simulink model "gazebo_cosimulation_waypoint_follower"  (R2023b)
settings: Solver=VariableStepAuto  StartTime=0.0  StopTime=10.0  RelTol=1e-3
undefined symbols (not defined in the file): center_cylinder, quadcopter, rotor_1, rotor_2, rotor_3, rotor_4
libraries: robotgazebolib x11, simulink x1
settings Model: Creator=rakshan  LastModifiedBy=rakshan

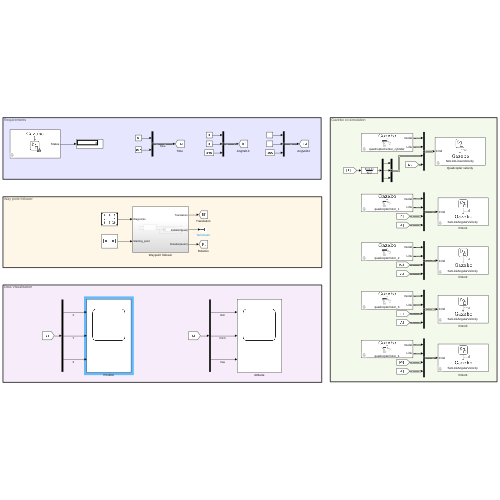
[thumbnail: Simulink's stored preview of the top-level diagram]
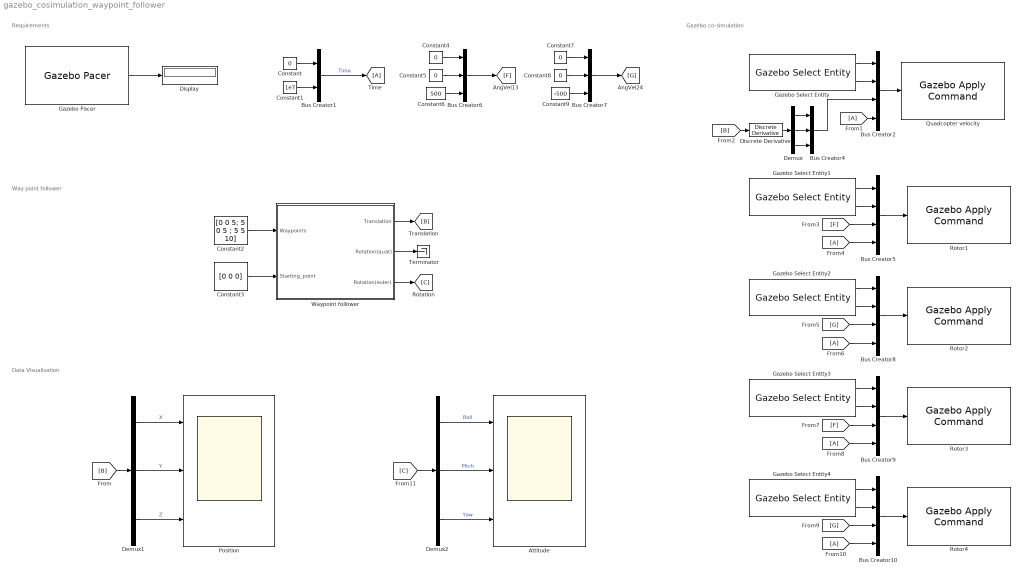
== system gazebo_cosimulation_waypoint_follower ==
  note: Data Visualisation
  note: Way point follower
  note: Requirements
  note: Gazebo co-simulation
  Attitude : Scope  NumInputPorts=3
  Bus Creator1 : BusCreator  Inputs=2  OutDataTypeStr=Bus: Gazebo_SL_Bus_gazebo_msgs_Time  NonVirtualBus=on
      settings: InheritFromInputs=off
  Bus Creator{5,8..10} (4 alike) : BusCreator  Inputs=4  OutDataTypeStr=Bus: Gazebo_SL_Bus_gazebo_msgs_SetLinkAngularVelocity  NonVirtualBus=on
      settings: InheritFromInputs=off
  Bus Creator2 : BusCreator  Inputs=4  OutDataTypeStr=Bus: Gazebo_SL_Bus_gazebo_msgs_SetLinkLinearVelocity  NonVirtualBus=on
      settings: InheritFromInputs=off
  Bus Creator4 : BusCreator  Inputs=3  OutDataTypeStr=Bus: Gazebo_SL_Bus_gazebo_msgs_Point  NonVirtualBus=on
      settings: InheritFromInputs=off
  Bus Creator6 : BusCreator  Inputs=3  OutDataTypeStr=Bus: Gazebo_SL_Bus_gazebo_msgs_Point  NonVirtualBus=on
      settings: InheritFromInputs=off
  Bus Creator7 : BusCreator  Inputs=3  OutDataTypeStr=Bus: Gazebo_SL_Bus_gazebo_msgs_Point  NonVirtualBus=on
      settings: InheritFromInputs=off
  Constant{,4..5,7..8} (5 alike) : Constant  Value=0
  Constant1 : Constant  Value=1e7
  Constant2 : Constant  Value=[0 0 5; 5 0 5 ; 5 5 10]
  Constant3 : Constant  Value=[0 0 0]  VectorParams1D=off
  Constant6 : Constant  Value=500
  Constant9 : Constant  Value=-500
  Demux : Demux  Outputs=3
  Demux1 : Demux  Outputs=3
  Demux2 : Demux  Outputs=3
  Discrete Derivative : simulink/Discrete/Discrete Derivative  gainval=1.0  ICPrevScaledInput=0.0  OutMin=[]  OutMax=[]  OutDataType=fixdt(1, 16)  OutScaling=2^-10  DoSatur=off
  Display : Display
  From{1,4,6,8,10} (5 alike) : From
  Gazebo Pacer : robotgazebolib/Gazebo Pacer  ResetBehavior=Reset Gazebo simulation time  SampleTime=0.001
  Gazebo Select Entity : robotgazebolib/Gazebo Select Entity  modelElemName=quadcopter/center_cylinder  outputArraySize=128  OutputLabel=Link  SelectType=Link
  Gazebo Select Entity1 : robotgazebolib/Gazebo Select Entity  modelElemName=quadcopter/rotor_1  outputArraySize=128  OutputLabel=Link  SelectType=Link
  Gazebo Select Entity2 : robotgazebolib/Gazebo Select Entity  modelElemName=quadcopter/rotor_2  outputArraySize=128  OutputLabel=Link  SelectType=Link
  Gazebo Select Entity3 : robotgazebolib/Gazebo Select Entity  modelElemName=quadcopter/rotor_3  outputArraySize=128  OutputLabel=Link  SelectType=Link
  Gazebo Select Entity4 : robotgazebolib/Gazebo Select Entity  modelElemName=quadcopter/rotor_4  outputArraySize=128  OutputLabel=Link  SelectType=Link
  Position : Scope  NumInputPorts=3
  Quadcopter velocity : robotgazebolib/Gazebo Apply Command  cmdType=SetLinkLinearVelocity  sampleTime=0.001
  Rotor{1..4} (4 alike) : robotgazebolib/Gazebo Apply Command  cmdType=SetLinkAngularVelocity  sampleTime=0.001
  Terminator : Terminator
  Time : Goto
  Waypoint follower : Subsystem
  wires:
  Constant3/1 -> Waypoint follower/2(Starting_point)
  Constant2/1 -> Waypoint follower/1(Waypoints)
  Waypoint follower/2(Rotation(quat)) -> Terminator/1
  Waypoint follower/1(Translation) -> [B]
  Waypoint follower/3(Rotation(euler)) -> [C]
  Bus Creator6/1 -> [F]
  Bus Creator1/1 -> Time/1  "Time"
  Constant5/1 -> Bus Creator6/2
  Constant4/1 -> Bus Creator6/1
  Constant6/1 -> Bus Creator6/3
  Constant9/1 -> Bus Creator7/3
  Constant8/1 -> Bus Creator7/2
  Gazebo Pacer/1 -> Display/1
  Constant/1 -> Bus Creator1/1
  Constant1/1 -> Bus Creator1/2
  Constant7/1 -> Bus Creator7/1
  Bus Creator7/1 -> [G]
  Gazebo Select Entity3/2 -> Bus Creator9/2
  Gazebo Select Entity1/1 -> Bus Creator5/1
  Bus Creator5/1 -> Rotor1/1
  Demux/3 -> Bus Creator4/3
  Gazebo Select Entity/2 -> Bus Creator2/2
  Demux/1 -> Bus Creator4/1
  [G] -> Bus Creator8/3
  Gazebo Select Entity/1 -> Bus Creator2/1
  From8/1 -> Bus Creator9/4
  [F] -> Bus Creator9/3
  Demux/2 -> Bus Creator4/2
  Gazebo Select Entity2/2 -> Bus Creator8/2
  From6/1 -> Bus Creator8/4
  [F] -> Bus Creator5/3
  Bus Creator2/1 -> Quadcopter velocity/1
  Bus Creator8/1 -> Rotor2/1
  Bus Creator4/1 -> Bus Creator2/3
  Bus Creator10/1 -> Rotor4/1
  From4/1 -> Bus Creator5/4
  From1/1 -> Bus Creator2/4
  Gazebo Select Entity4/2 -> Bus Creator10/2
  Gazebo Select Entity4/1 -> Bus Creator10/1
  Gazebo Select Entity1/2 -> Bus Creator5/2
  Gazebo Select Entity3/1 -> Bus Creator9/1
  [G] -> Bus Creator10/3
  Gazebo Select Entity2/1 -> Bus Creator8/1
  Bus Creator9/1 -> Rotor3/1
  From10/1 -> Bus Creator10/4
  [B] -> Discrete Derivative/1
  Discrete Derivative/1 -> Demux/1
  Demux1/1 -> Position/1  "X"
  Demux1/2 -> Position/2  "Y"
  Demux1/3 -> Position/3  "Z"
  Demux2/1 -> Attitude/1  "Roll"
  Demux2/2 -> Attitude/2  "Pitch"
  Demux2/3 -> Attitude/3  "Yaw"
  [B] -> Demux1/1
  [C] -> Demux2/1

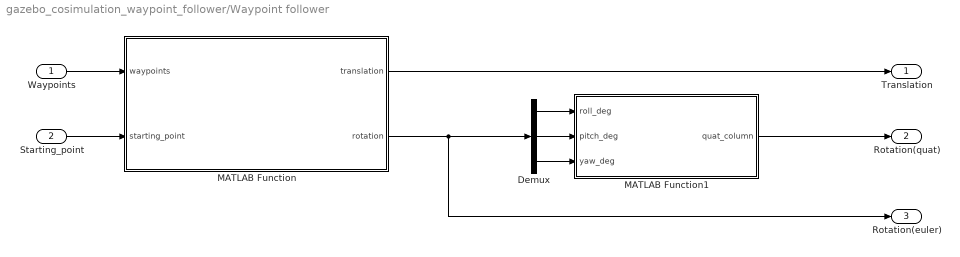
== system gazebo_cosimulation_waypoint_follower/Waypoint follower ==
  Waypoints : Inport
  Starting_point : Inport  Port=2
  Demux : Demux  Outputs=3
  MATLAB Function : MATLAB Function  TreatAsAtomicUnit=on
  MATLAB Function1 : MATLAB Function  TreatAsAtomicUnit=on
  Translation : Outport
  Rotation(quat) : Outport  Port=2
  Rotation(euler) : Outport  Port=3
  wires:
  Demux/1 -> MATLAB Function1/1(roll_deg)
  Demux/3 -> MATLAB Function1/3(yaw_deg)
  Demux/2 -> MATLAB Function1/2(pitch_deg)
  MATLAB Function1/1(quat_column) -> Rotation(quat)/1
  MATLAB Function/2(rotation) -> Rotation(euler)/1, Demux/1
  Waypoints/1 -> MATLAB Function/1(waypoints)
  Starting_point/1 -> MATLAB Function/2(starting_point)
  MATLAB Function/1(translation) -> Translation/1

== matlab function gazebo_cosimulation_waypoint_follower/Waypoint follower/MATLAB Function ==
  data: waypoints input; translation output; rotation output; starting_point input
function [translation, rotation] = interpolateWaypointsSimulink(waypoints,starting_point)
    persistent current_waypoint;
    persistent current_index;
    time_step = 0.002;
   
    waypoints = [starting_point;waypoints]
    % Initialize persistent variables on first call
    if isempty(current_waypoint)
        current_waypoint = waypoints(1,:);
        current_index = 1;
    end
    
    % Initialize outputs
    translation = zeros(1, 3);
    rotation = zeros(1, 3); % Euler angles: [yaw, pitch, roll]
    
    % Check if reached last waypoint
    if current_index == size(waypoints, 1)
        translation = waypoints(end, :);
        rotation = [0 0 0]; % No rotation (identity)
    else
        % Interpolate translation
        translation = current_waypoint;
        next_waypoint = waypoints(current_index + 1, :);
        current_waypoint = current_waypoint + (next_waypoint - current_waypoint) * time_step;
        
        % Calculate direction vector
        direction_vector = next_waypoint - current_waypoint;
        direction_vector = direction_vector / norm(direction_vector); % Normalize
        
        % Calculate rotation angles (Euler angles)
        yaw = atan2(direction_vector(2), direction_vector(1));
        pitch = asin(direction_vector(3));
        roll = 0; % Assuming no roll motion
        
        % Update rotation
        rotation = [yaw pitch roll];
        
        % Check if reached next waypoint
        if norm(current_waypoint - next_waypoint) < 0.01
            current_index = current_index + 1;
        end
    end
end

== matlab function gazebo_cosimulation_waypoint_follower/Waypoint follower/MATLAB Function1 ==
  data: roll_deg input; quat_column output; pitch_deg input; yaw_deg input
function quat_column = eulerToQuat(roll_deg, pitch_deg, yaw_deg)
    % Convert Euler angles to radians
    roll_rad = deg2rad(roll_deg);
    pitch_rad = deg2rad(pitch_deg);
    yaw_rad = deg2rad(yaw_deg);

    % Calculate half angles
    roll_half = roll_rad / 2;
    pitch_half = pitch_rad / 2;
    yaw_half = yaw_rad / 2;

    % Calculate trigonometric functions
    roll_sin = sin(roll_half);
    roll_cos = cos(roll_half);
    pitch_sin = sin(pitch_half);
    pitch_cos = cos(pitch_half);
    yaw_sin = sin(yaw_half);
    yaw_cos = cos(yaw_half);

    % Calculate quaternion components
    q0 = roll_cos * pitch_cos * yaw_cos + roll_sin * pitch_sin * yaw_sin;
    q1 = roll_sin * pitch_cos * yaw_cos - roll_cos * pitch_sin * yaw_sin;
    q2 = roll_cos * pitch_sin * yaw_cos + roll_sin * pitch_cos * yaw_sin;
    q3 = roll_cos * pitch_cos * yaw_sin - roll_sin * pitch_sin * yaw_cos;

    % Format the quaternion as a column vector
    quat_column = [q0; q1; q2; q3];
end
